simulink subsystem "thread"  (R2023b)
settings: Solver=VariableStepAuto  StartTime=0.0  StopTime=10.0  RelTol=1e-3
values from neighbouring files (symbols this model uses):
  spf_mat = 1024    [inizio.m]    (also in load_preset_audio.m)
settings Model: Creator=Edp  LastModifiedBy=giorg

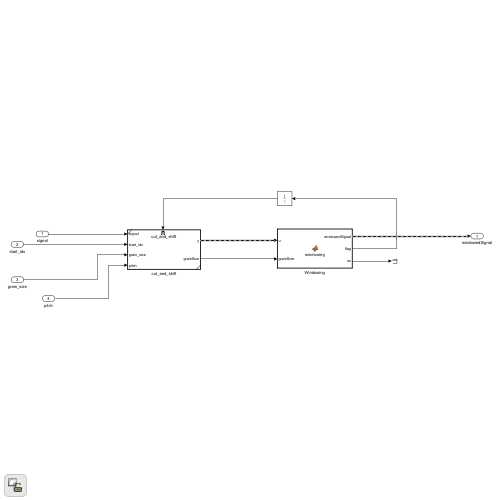
[thumbnail: Simulink's stored preview of the top-level diagram]
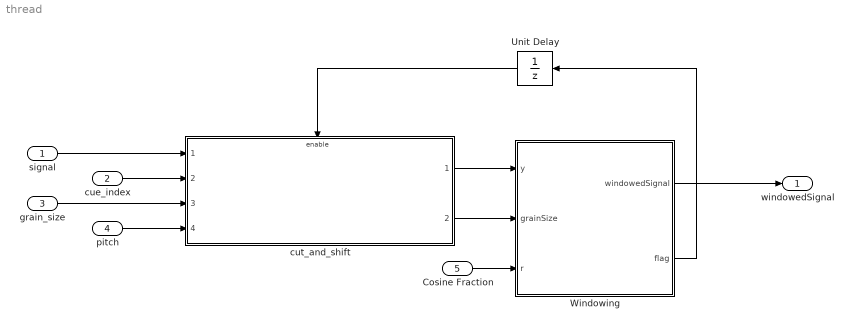
== system thread ==
  signal : Inport
  cue_index : Inport  Port=2
  grain_size : Inport  Port=3
  pitch : Inport  Port=4
  Cosine Fraction : Inport  Port=5
  Unit Delay : UnitDelay  InitialCondition=1  SampleTime=-1  HasFrameUpgradeWarning=on
  Windowing : MATLAB Function  TreatAsAtomicUnit=on  mask{spf=spf_mat}
  cut_and_shift : Subsystem  ReferencedSubsystem=cut_and_shift
  windowedSignal : Outport
  wires:
  Unit Delay/1 -> cut_and_shift/Enable
  grain_size/1 -> cut_and_shift/3
  cut_and_shift/1 -> Windowing/1(y)
  pitch/1 -> cut_and_shift/4
  Windowing/2(flag) -> Unit Delay/1
  Windowing/1(windowedSignal) -> windowedSignal/1
  signal/1 -> cut_and_shift/1
  cut_and_shift/2 -> Windowing/2(grainSize)
  cue_index/1 -> cut_and_shift/2
  Cosine Fraction/1 -> Windowing/3(r)

== matlab function thread/Windowing ==
  data: y input; grainSize input; windowedSignal output size=1024; spf parameter uint32 size=1; flag output; r input
% INPUT: extracted grain (y), size of the grain (grainSize), output audio
% buffer (spf), cosine fraction (r)

% OUTPUT: portion of the windowed signal of length spf (windowedSignal),
% flag that identifies the end of the grain

% If the grain size is not a multiple of spf, the function completes the
% buffer with the starting samples of the next grain

function [windowedSignal, flag] = windowing(y, grainSize, spf, r)
    % r is the cosine fraction: 
    % If r == 0 -> rectangular window
    % If r == 1 -> hann window
    windowSize = grainSize;
    % Initialize persistent variables
    persistent it window windowedBuffer grain sz;
    % Initialize flag and sz
    flag = 0;
    if isempty(grain)
        grain = 0;
    end
    % Check if it is the first call or window needs to be initialized
    if isempty(it) || isempty(window)
        it = 1; % Initialize iteration count
        window = tukeywin(windowSize, r); % Initialize window
    end
    
    if isempty(sz)
        sz = 0;
    end
    % Check if windowedBuffer needs to be initialized
    if isempty(windowedBuffer)
        windowedBuffer = -ones(1024, 1);
    end
    windowedBuffer(windowedBuffer == -1) = [];
    % Append the buffer from previous grain (if there is any)
    if it == 1
        grain = grainSize;
        window = tukeywin(grain, r);
        y = [windowedBuffer; y]; % Append buffer to the beginning of u
        windowedBuffer = [];
    end
    
    if it == 1 && sz == 0
        startIndex = (it - 1) * spf + 1; % 1
        endIndex = startIndex + spf - 1; % 1024
        windowedSignal = y(startIndex:endIndex) .* window(startIndex:endIndex);
    elseif it == 1 && sz ~= 0
        startIndex = uint32((it - 1) * spf + 1); % 1
        endIndex = uint32(startIndex + spf - 1); % 1024
        windowedSignal = [y(startIndex:startIndex + sz - 1);y((startIndex + sz):endIndex) .* window(startIndex:(endIndex - sz))];
    else
        startIndex = (it - 1) * spf + 1 - sz;
        endIndex = startIndex + spf - 1;
        windowedSignal = y(startIndex:endIndex) .* window(startIndex:endIndex);
    end
    

    % Increment the iteration count
    it = it + 1;
    % Check if we've reached the end of the window
    if (it * spf - sz) >= grain
        % Reset the iteration count
        it = 1;
        % Store the remaining samples for the next iteration
        windowedBuffer = y(endIndex + 1:end) .* window(endIndex + 1:end);
        sz = size(windowedBuffer, 1);
        % Set the flag to indicate the end of the grain
        flag = 1;
    end
end
